simulink library "copterFtc_lib"  (R2018b)
settings: Solver=VariableStepAuto  StartTime=0.0  StopTime=10.0  RelTol=1e-3
undefined symbols (not defined in the file or in its folder): DiscIntNeverNeededParam, fm_loiter, simin
libraries: simulink x2, fmCopterAltHoldIndi_lib x2, cntrlAttiRedIndi_lib x2, indi_lib x1, control_allocation_lib x1, ndi_lib x1, filters_lib x1, cntrlPosNdi_lib x1, axes_transformation_lib x1
settings Model: Creator=Ybeyer  LastModifiedBy=yannic
settings SFSimCC: SimUseLocalCustomCode=off
settings RTWCC: RTWUseLocalCustomCode=off
settings CodeAppCC: StateflowObjectComments=on

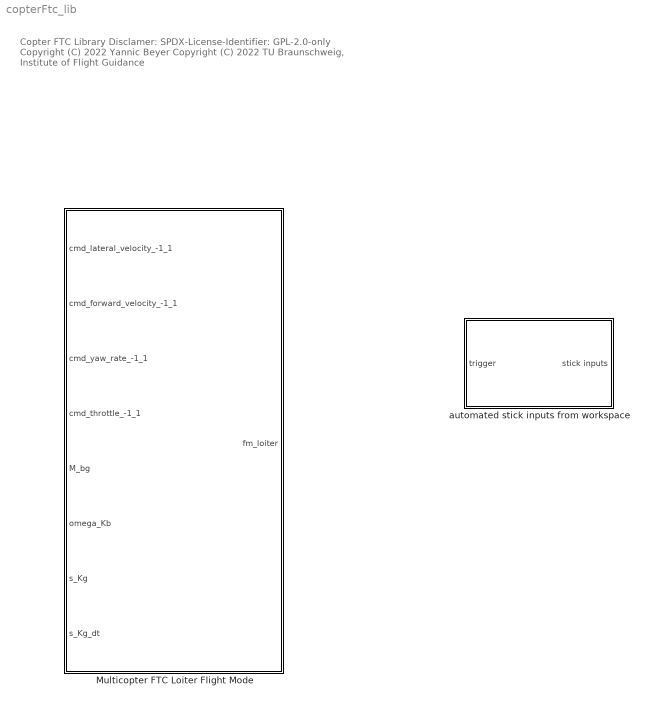
== system copterFtc_lib ==
  note: Copter FTC Library
      |
      | Disclamer:
      | SPDX-License-Identifier: GPL-2.0-only
      |
      | Copyright (C) 2022 Yannic Beyer
      | Copyright (C) 2022 TU Braunschweig, Institute of Flight Guidance
  Multicopter FTC Loiter Flight Mode : Subsystem  mask{fm=fm_loiter}
      mask prompts: fm "Multicopter INDI loiter flight  struct"
      mask DialogControl DescGroupVar Prompt: Multicopter INDI Loiter Flight Mode
      mask DialogControl DescTextVar Prompt: Loiter flight mode using the reduced attitude controller with INDI.
      mask DialogControl Control2 Prompt: To intialize the parameters struct see multicopterFlightModeLoiter.
  automated stick inputs from workspace : Subsystem  mask{simin=simin}
      mask prompts: simin "simin struct"
      mask DialogControl DescGroupVar Prompt: Automated stick inputs from workspace
      mask DialogControl DescTextVar Prompt: The stick inputs must be defined as a struct for the standard block "from workspace".

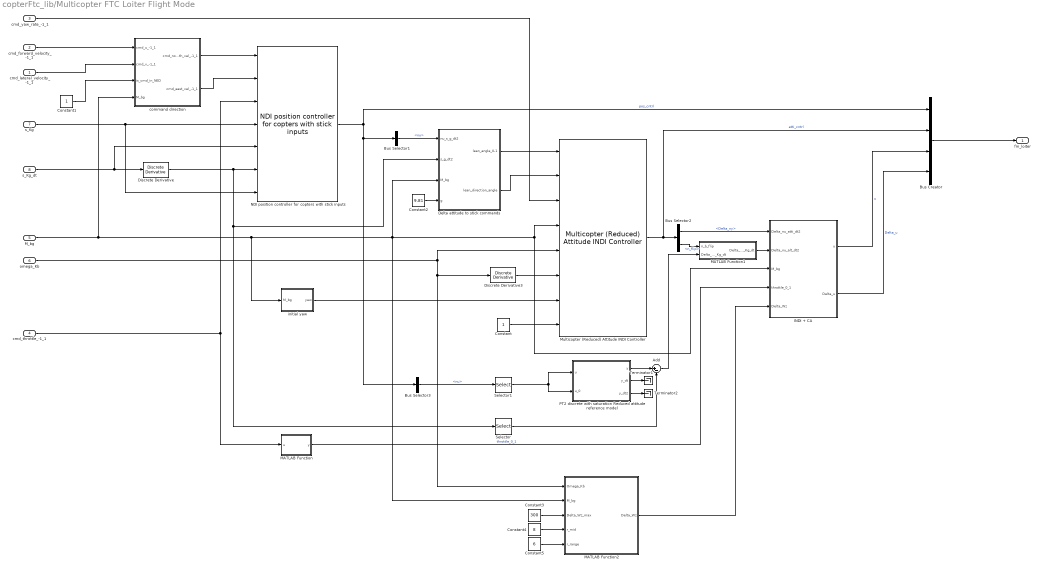
== system copterFtc_lib/Multicopter FTC Loiter Flight Mode ==
  cmd_lateral_velocity_-1_1 : Inport  SampleTime=fm.sample_time
  cmd_forward_velocity_-1_1 : Inport  Port=2  SampleTime=fm.sample_time
  cmd_yaw_rate_-1_1 : Inport  Port=3  SampleTime=fm.sample_time
  cmd_throttle_-1_1 : Inport  Port=4  SampleTime=fm.sample_time
  M_bg : Inport  Port=5  SampleTime=fm.sample_time
  omega_Kb : Inport  Port=6  SampleTime=fm.sample_time
  s_Kg : Inport  Port=7  SampleTime=fm.sample_time
  s_Kg_dt : Inport  Port=8  SampleTime=fm.sample_time
  Add : Sum  Inputs=|+-
  Bus Creator : BusCreator  Inputs=4
  Bus Selector1 : BusSelector  OutputSignals=pseudo_control.nu
  Bus Selector2 : BusSelector  OutputSignals=pseudo_control.Delta_ny,reference.reduced_attitude.n_flip
  Bus Selector3 : BusSelector  OutputSignals=pseudo_control.nu
  Constant : Constant
  Constant1 : Constant
  Constant2 : Constant  Value=9.81
  Constant3 : Constant  Value=300
  Constant4 : Constant  Value=8
  Constant5 : Constant  Value=6
  Delta attitude to stick commands : Subsystem
  Discrete Derivative : simulink/Discrete/Discrete Derivative  gainval=1.0  ICPrevScaledInput=0.0  OutMin=[]  OutMax=[]  OutDataType=fixdt(1, 16)  OutScaling=2^-10  DoSatur=off
  Discrete Derivative3 : simulink/Discrete/Discrete Derivative  gainval=1.0  ICPrevScaledInput=0.0  OutMin=[]  OutMax=[]  OutDataType=fixdt(1, 16)  OutScaling=2^-10  DoSatur=off
  INDI + CA : Subsystem
  MATLAB Function : MATLAB Function  TreatAsAtomicUnit=on
  MATLAB Function1 : MATLAB Function  TreatAsAtomicUnit=on
  MATLAB Function2 : MATLAB Function  TreatAsAtomicUnit=on
  Multicopter (Reduced) Attitude INDI Controller : cntrlAttiRedIndi_lib/Multicopter (Reduced) Attitude INDI Controller  atc=fm.atc  T=fm.motor_time_constant + 2./fm.sens_filt.omega
  NDI position controller for copters with stick inputs : cntrlPosNdi_lib/NDI position controller for copters with stick inputs  psc=fm.psc  T_inner_loop=2./fm.atc.rm.leanfreq + fm.motor_time_constant + 2./fm.sens_filt.omega
      settings: SourceProductName=LADAC
  PT2 discrete with saturation Reduced attitude reference model : Subsystem  mask{omega=fm.atc.rm.leanfreq, d=fm.atc.rm.leandamp, x_dt2_max=inf, x_dt2_min=-inf, x_dt_max=inf, x_dt_min=-inf, x_max=inf, x_min=-inf, x_init=0, x_dt_init=0}
      mask prompts: omega "Natural frequency"; d "Damping ratio"; x_dt2_max "Maximum acceleration"; x_dt2_min "Minimum acceleration"; x_dt_max "Maximum rate"; x_dt_min "Minimum rate"; x_max "Maximum position"; x_min "Minimum position"; x_init "Initial position"; x_dt_init "Initial rate"
  Selector : Selector  InputPortWidth=3  IndexOptions=Index vector (dialog)  Indices=3  OutputSizes=1
  Selector1 : Selector  InputPortWidth=3  IndexOptions=Index vector (dialog)  Indices=3  OutputSizes=1
  Terminator1 : Terminator
  Terminator2 : Terminator
  command direction : Subsystem
  initial yaw : Subsystem
  fm_loiter : Outport  SampleTime=fm.sample_time
  wires:
  cmd_forward_velocity_-1_1/1 -> command direction/1(cmd_u_-1_1)
  s_Kg_dt/1 -> NDI position controller for copters with stick inputs/5, Discrete Derivative/1
  Discrete Derivative/1 -> Selector/1, Delta attitude to stick commands/2(s_g_dt2), NDI position controller for copters with stick inputs/6
  cmd_yaw_rate_-1_1/1 -> Multicopter (Reduced) Attitude INDI Controller/3
  Constant/1 -> Multicopter (Reduced) Attitude INDI Controller/8
  s_Kg/1 -> NDI position controller for copters with stick inputs/7, NDI position controller for copters with stick inputs/4
  omega_Kb/1 -> MATLAB Function2/1(Omega_Kb), Discrete Derivative3/1, Multicopter (Reduced) Attitude INDI Controller/5
  NDI position controller for copters with stick inputs/1 -> Bus Selector3/1, Bus Selector1/1, Bus Creator/1  "pos_cntrl"
  M_bg/1 -> command direction/4(M_bg), MATLAB Function2/2(M_bg), Multicopter (Reduced) Attitude INDI Controller/4, INDI + CA/3(M_bg), Delta attitude to stick commands/3(M_bg), initial yaw/1(M_bg)
  cmd_lateral_velocity_-1_1/1 -> command direction/2(cmd_v_-1_1)
  Constant1/1 -> command direction/3(is_cmd_in_NED)
  Bus Selector1/1 -> Delta attitude to stick commands/1(nu_s_g_dt2)  "<nu>"
  Bus Creator/1 -> fm_loiter/1
  command direction/1(cmd_north_vel_-1_1) -> NDI position controller for copters with stick inputs/1
  command direction/2(cmd_east_vel_-1_1) -> NDI position controller for copters with stick inputs/2
  Multicopter (Reduced) Attitude INDI Controller/1 -> Bus Selector2/1, Bus Creator/2  "atti_cntrl"
  Bus Selector3/1 -> Selector1/1  "<nu>"
  Discrete Derivative3/1 -> Multicopter (Reduced) Attitude INDI Controller/6
  Delta attitude to stick commands/2(lean_direction_angle) -> Multicopter (Reduced) Attitude INDI Controller/2
  Delta attitude to stick commands/1(lean_angle_0-1) -> Multicopter (Reduced) Attitude INDI Controller/1
  MATLAB Function/1(y) -> INDI + CA/4(throttle_0_1)  "throttle_0_1"
  INDI + CA/1(u) -> Bus Creator/3  "u"
  INDI + CA/2(Delta_u) -> Bus Creator/4  "Delta_u"
  cmd_throttle_-1_1/1 -> NDI position controller for copters with stick inputs/3, MATLAB Function/1(u)
  Bus Selector2/1 -> INDI + CA/1(Delta_nu_atti_dt2)  "<Delta_ny>"
  MATLAB Function1/1(Delta_nu_w_Kg_dt) -> INDI + CA/2(Delta_nu_alt_dt2)
  Bus Selector2/2 -> MATLAB Function1/1(n_b_flip)  "<n_flip>"
  Constant2/1 -> Delta attitude to stick commands/4(g)
  Selector/1 -> Add/2
  PT2 discrete with saturation Reduced attitude reference model/2(y_dt) -> Terminator1/1
  PT2 discrete with saturation Reduced attitude reference model/3(y_dt2) -> Terminator2/1
  Selector1/1 -> PT2 discrete with saturation Reduced attitude reference model/1(u), PT2 discrete with saturation Reduced attitude reference model/2(u_0)
  Add/1 -> MATLAB Function1/2("Delta_nu_w_Kg_dt ")
  PT2 discrete with saturation Reduced attitude reference model/1(y) -> Add/1
  MATLAB Function2/1(Delta_Wz) -> INDI + CA/5(Delta_Wz)
  Constant3/1 -> MATLAB Function2/3(Delta_Wz_max)
  Constant4/1 -> MATLAB Function2/4(r_mid)
  Constant5/1 -> MATLAB Function2/5(r_range)
  initial yaw/1(yaw) -> Multicopter (Reduced) Attitude INDI Controller/7

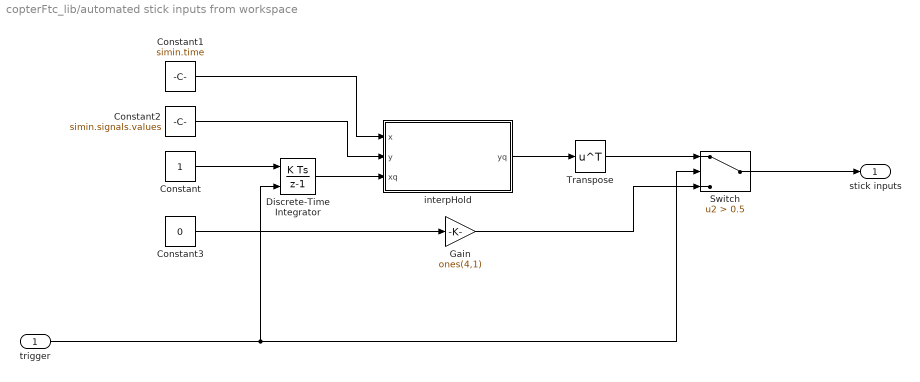
== system copterFtc_lib/automated stick inputs from workspace ==
  trigger : Inport
  Constant : Constant
  Constant1 : Constant  Value=simin.time
  Constant2 : Constant  Value=simin.signals.values
  Constant3 : Constant  Value=0
  Discrete-Time Integrator : DiscreteIntegrator  ExternalReset=rising  SampleTime=-1  ICPrevOutput=DiscIntNeverNeededParam  ICPrevScaledInput=DiscIntNeverNeededParam
  Gain : Gain  Gain=ones(4,1)
  Switch : Switch  Criteria=u2 > Threshold  Threshold=0.5
  Transpose : Math  Operator=transpose  SaturateOnIntegerOverflow=on
  interpHold : MATLAB Function  TreatAsAtomicUnit=on
  stick inputs : Outport
  wires:
  Constant1/1 -> interpHold/1(x)
  Discrete-Time Integrator/1 -> interpHold/3(xq)
  interpHold/1(yq) -> Transpose/1
  Constant2/1 -> interpHold/2(y)
  Constant/1 -> Discrete-Time Integrator/1
  Constant3/1 -> Gain/1
  Switch/1 -> stick inputs/1
  Gain/1 -> Switch/3
  Transpose/1 -> Switch/1
  trigger/1 -> Switch/2, Discrete-Time Integrator/2

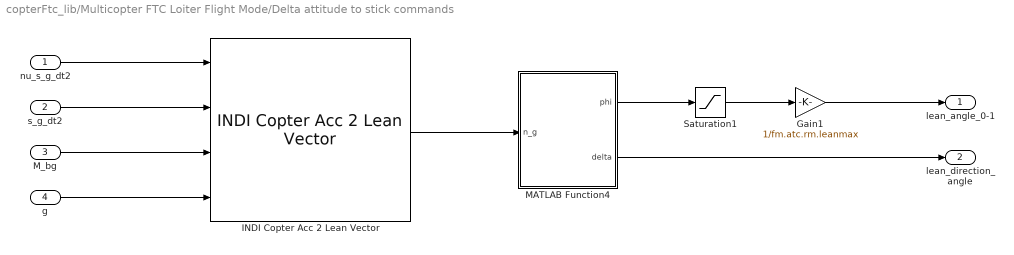
== system copterFtc_lib/Multicopter FTC Loiter Flight Mode/Delta attitude to stick commands ==
  nu_s_g_dt2 : Inport
  s_g_dt2 : Inport  Port=2
  M_bg : Inport  Port=3
  g : Inport  Port=4
  Gain1 : Gain  Gain=1/fm.atc.rm.leanmax
  INDI Copter Acc 2 Lean Vector : indi_lib/INDI Copter Acc 2 Lean Vector  SystemSampleTime=-1
      settings: SourceProductName=LADAC
  MATLAB Function4 : MATLAB Function  TreatAsAtomicUnit=on
  Saturation1 : Saturate  UpperLimit=fm.atc.rm.leanmax  LowerLimit=0
  lean_angle_0-1 : Outport
  lean_direction_angle : Outport  Port=2
  wires:
  M_bg/1 -> INDI Copter Acc 2 Lean Vector/3
  s_g_dt2/1 -> INDI Copter Acc 2 Lean Vector/2
  g/1 -> INDI Copter Acc 2 Lean Vector/4
  MATLAB Function4/1(phi) -> Saturation1/1
  Saturation1/1 -> Gain1/1
  nu_s_g_dt2/1 -> INDI Copter Acc 2 Lean Vector/1
  Gain1/1 -> lean_angle_0-1/1
  MATLAB Function4/2(delta) -> lean_direction_angle/1
  INDI Copter Acc 2 Lean Vector/1 -> MATLAB Function4/1(n_g)

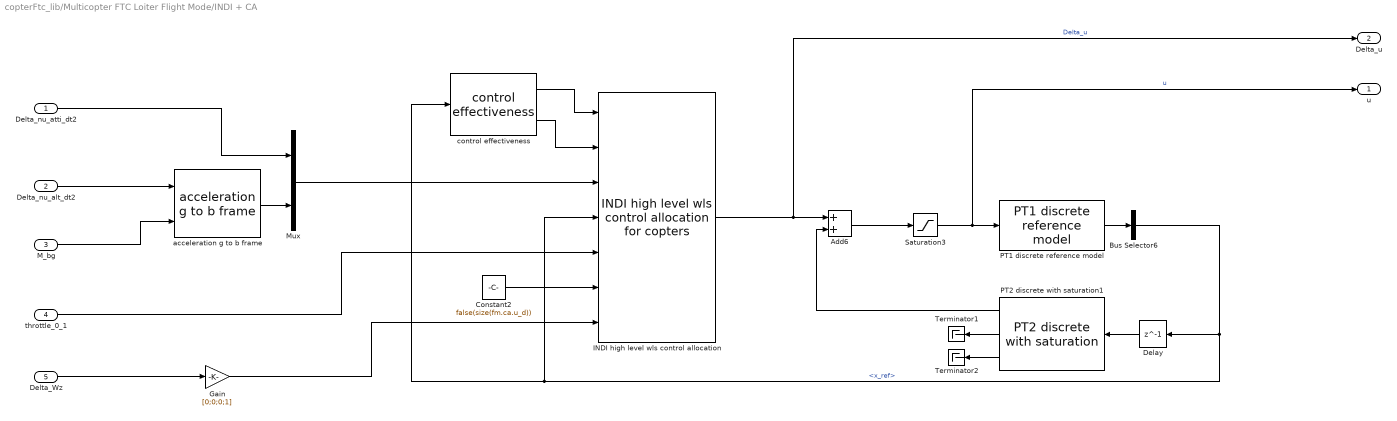
== system copterFtc_lib/Multicopter FTC Loiter Flight Mode/INDI + CA ==
  Delta_nu_atti_dt2 : Inport
  Delta_nu_alt_dt2 : Inport  Port=2
  M_bg : Inport  Port=3
  throttle_0_1 : Inport  Port=4
  Delta_Wz : Inport  Port=5
  Add6 : Sum
  Bus Selector6 : BusSelector  OutputSignals=x_ref
  Constant2 : Constant  Value=false(size(fm.ca.u_d))
  Delay : Delay  DelayLength=1
  Gain : Gain  Gain=[0;0;0;1]
  INDI high level wls control allocation : control_allocation_lib/INDI high level wls control allocation for copters  ca=fm.ca  is_Delta_W_v_check=on  is_W_check=off  is_iter_check=off
  Mux : Mux  Inputs=2
  PT1 discrete reference model : ndi_lib/PT1 discrete reference model  T=fm.motor_time_constant  x_max=inf  x_min=-inf  x_dt_max=inf  x_dt_min=-inf  x_init=0
      settings: SourceProductName=LADAC
  PT2 discrete with saturation1 : filters_lib/PT2 discrete with saturation  omega=fm.sens_filt.omega  d=fm.sens_filt.D  x_dt2_max=inf  x_dt2_min=-inf  x_dt_max=inf  x_dt_min=-inf  x_max=inf  x_min=-inf  x_init=0  x_dt_init=0
      settings: SourceProductName=LADAC
  Saturation3 : Saturate  UpperLimit=fm.ca.u_max  LowerLimit=fm.ca.u_min
  Terminator1 : Terminator
  Terminator2 : Terminator
  acceleration g to b frame : fmCopterAltHoldIndi_lib/Multicopter Altitude Hold Flight Mode with INDI and reduced attitude control/acceleration g to b frame  SystemSampleTime=-1
      settings: SourceProductName=LADAC
  control effectiveness : fmCopterAltHoldIndi_lib/Multicopter Altitude Hold Flight Mode with INDI and reduced attitude control/control effectiveness  SystemSampleTime=-1
      settings: SourceProductName=LADAC
  u : Outport
  Delta_u : Outport  Port=2
  wires:
  PT2 discrete with saturation1/1 -> Add6/2
  Mux/1 -> INDI high level wls control allocation/3
  Saturation3/1 -> u/1, PT1 discrete reference model/1  "u"
  INDI high level wls control allocation/1 -> Delta_u/1, Add6/1  "Delta_u"
  Delay/1 -> PT2 discrete with saturation1/1
  throttle_0_1/1 -> INDI high level wls control allocation/5
  Bus Selector6/1 -> Delay/1, control effectiveness/1, INDI high level wls control allocation/4  "<x_ref>"
  control effectiveness/1 -> INDI high level wls control allocation/1
  Constant2/1 -> INDI high level wls control allocation/6
  PT2 discrete with saturation1/2 -> Terminator1/1
  PT2 discrete with saturation1/3 -> Terminator2/1
  PT1 discrete reference model/1 -> Bus Selector6/1
  Add6/1 -> Saturation3/1
  Delta_nu_atti_dt2/1 -> Mux/1
  acceleration g to b frame/1 -> Mux/2
  Delta_nu_alt_dt2/1 -> acceleration g to b frame/1
  M_bg/1 -> acceleration g to b frame/2
  control effectiveness/2 -> INDI high level wls control allocation/2
  Delta_Wz/1 -> Gain/1
  Gain/1 -> INDI high level wls control allocation/7

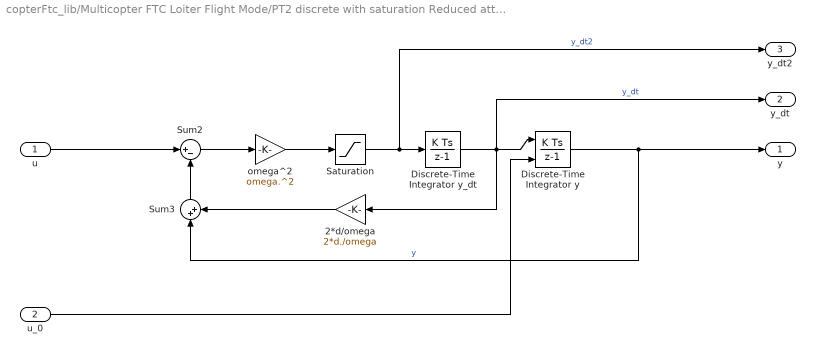
== system copterFtc_lib/Multicopter FTC Loiter Flight Mode/PT2 discrete with saturation Reduced attitude reference model ==
  u : Inport
  u_0 : Inport  Port=2
  2*d/omega : Gain  Gain=2*d./omega
  Discrete-Time Integrator y : DiscreteIntegrator  InitialConditionSource=external  InitialCondition=x_init  SampleTime=-1  OutDataTypeStr=Inherit: Inherit via back propagation  LimitOutput=on  UpperSaturationLimit=x_max  LowerSaturationLimit=x_min  ICPrevOutput=DiscIntNeverNeededParam  ICPrevScaledInput=DiscIntNeverNeededParam
  Discrete-Time Integrator y_dt : DiscreteIntegrator  InitialCondition=x_dt_init  SampleTime=-1  OutDataTypeStr=Inherit: Inherit via back propagation  LimitOutput=on  UpperSaturationLimit=x_dt_max  LowerSaturationLimit=x_dt_min  ICPrevOutput=DiscIntNeverNeededParam  ICPrevScaledInput=DiscIntNeverNeededParam
  Saturation : Saturate  UpperLimit=x_dt2_max  LowerLimit=x_dt2_min
  Sum2 : Sum  Inputs=|+-
  Sum3 : Sum  Inputs=|++
  omega^2 : Gain  Gain=omega.^2
  y : Outport
  y_dt : Outport  Port=2
  y_dt2 : Outport  Port=3
  wires:
  u_0/1 -> Discrete-Time Integrator y/2
  Discrete-Time Integrator y_dt/1 -> Discrete-Time Integrator y/1, y_dt/1, 2*d/omega/1  "y_dt"
  Discrete-Time Integrator y/1 -> y/1, Sum3/1  "y"
  Sum2/1 -> omega^2/1
  2*d/omega/1 -> Sum3/2
  u/1 -> Sum2/1
  Sum3/1 -> Sum2/2
  omega^2/1 -> Saturation/1
  Saturation/1 -> Discrete-Time Integrator y_dt/1, y_dt2/1  "y_dt2"

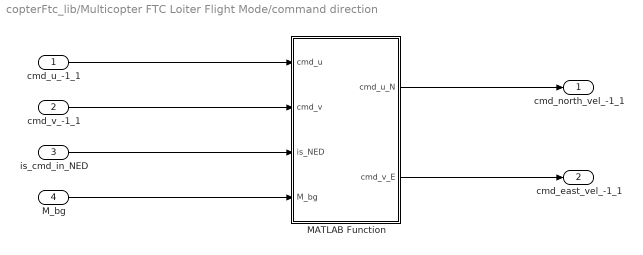
== system copterFtc_lib/Multicopter FTC Loiter Flight Mode/command direction ==
  cmd_u_-1_1 : Inport
  cmd_v_-1_1 : Inport  Port=2
  is_cmd_in_NED : Inport  Port=3
  M_bg : Inport  Port=4
  MATLAB Function : MATLAB Function  TreatAsAtomicUnit=on
  cmd_north_vel_-1_1 : Outport
  cmd_east_vel_-1_1 : Outport  Port=2
  wires:
  cmd_u_-1_1/1 -> MATLAB Function/1(cmd_u)
  cmd_v_-1_1/1 -> MATLAB Function/2(cmd_v)
  is_cmd_in_NED/1 -> MATLAB Function/3(is_NED)
  MATLAB Function/1(cmd_u_N) -> cmd_north_vel_-1_1/1
  MATLAB Function/2(cmd_v_E) -> cmd_east_vel_-1_1/1
  M_bg/1 -> MATLAB Function/4(M_bg)

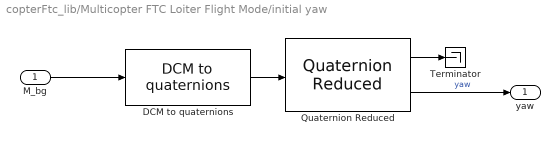
== system copterFtc_lib/Multicopter FTC Loiter Flight Mode/initial yaw ==
  M_bg : Inport
  DCM to quaternions : axes_transformation_lib/DCM to quaternions  SystemSampleTime=-1
      settings: SourceProductName=LADAC
  Quaternion Reduced : cntrlAttiRedIndi_lib/Multicopter (Reduced) Attitude INDI Controller/measure/Quaternion Reduced  SystemSampleTime=-1
  Terminator : Terminator
  yaw : Outport
  wires:
  DCM to quaternions/1 -> Quaternion Reduced/1
  M_bg/1 -> DCM to quaternions/1
  Quaternion Reduced/2 -> yaw/1  "yaw"
  Quaternion Reduced/1 -> Terminator/1

== matlab function copterFtc_lib/Multicopter FTC Loiter Flight Mode/command direction/MATLAB Function ==
  data: cmd_u input; cmd_u_N output; cmd_v input; is_NED input; cmd_v_E output; M_bg input
function [cmd_u_N,cmd_v_E] = fcn( cmd_u, cmd_v, is_NED, M_bg )

if is_NED
    cmd_u_N = cmd_u;
    cmd_v_E = cmd_v;
else
    EulerAngle = dcm2Euler(M_bg);
    yaw = EulerAngle(3);
    M_NED_FRD = euler2Dcm([0;0;yaw])';
    cmd_V_NED = M_NED_FRD * [ cmd_u; cmd_v; 0 ];
    cmd_u_N = cmd_V_NED(1);
    cmd_v_E = cmd_V_NED(2);
end

end

== matlab function copterFtc_lib/Multicopter FTC Loiter Flight Mode/MATLAB Function1 ==
  data: n_b_flip input; Delta_nu_w_Kg_dt input; Delta_nu_w_Kg_dt output
function Delta_nu_w_Kg_dt = fcn( n_b_flip, Delta_nu_w_Kg_dt )

if n_b_flip(3) >= 0
    Delta_nu_w_Kg_dt(:) = 0;
end

end

== matlab function copterFtc_lib/Multicopter FTC Loiter Flight Mode/Delta attitude to stick commands/MATLAB Function4 ==
  data: n_g input; phi output; delta output
function [phi,delta] = leanVector2LeanAngles(n_g)
[phi,delta] = leanVector2LeanAngles(n_g);
end

== matlab function copterFtc_lib/Multicopter FTC Loiter Flight Mode/MATLAB Function ==
  data: u input; y output
function y = fcn(u)
y = 0.5*u+0.5;

== matlab function copterFtc_lib/Multicopter FTC Loiter Flight Mode/MATLAB Function2 ==
  data: Omega_Kb input; Delta_Wz output; M_bg input; Delta_Wz_max input; r_mid input; r_range input
function Delta_Wz = caWlsDeltaWz( Omega_Kb, M_bg, Delta_Wz_max, r_mid, r_range )
Delta_Wz = caWlsDeltaWz( Omega_Kb, M_bg, Delta_Wz_max, r_mid, r_range );
end

== matlab function copterFtc_lib/automated stick inputs from workspace/interpHold ==
  data: x input; yq output; y input; xq input
function yq = interpHold( x, y, xq )
yq = interpHold( x, y, xq );
end
